simulink model "test_loopback_mux"  (Simulink 7.0)
settings: Solver=ode45  StartTime=0.0  StopTime=4000  RelTol=1e-3
libraries: xbsIndex_r4 x498, xps_library x21, xbsReplacements_r4 x18, casper_library x15
(part 2 of 3)

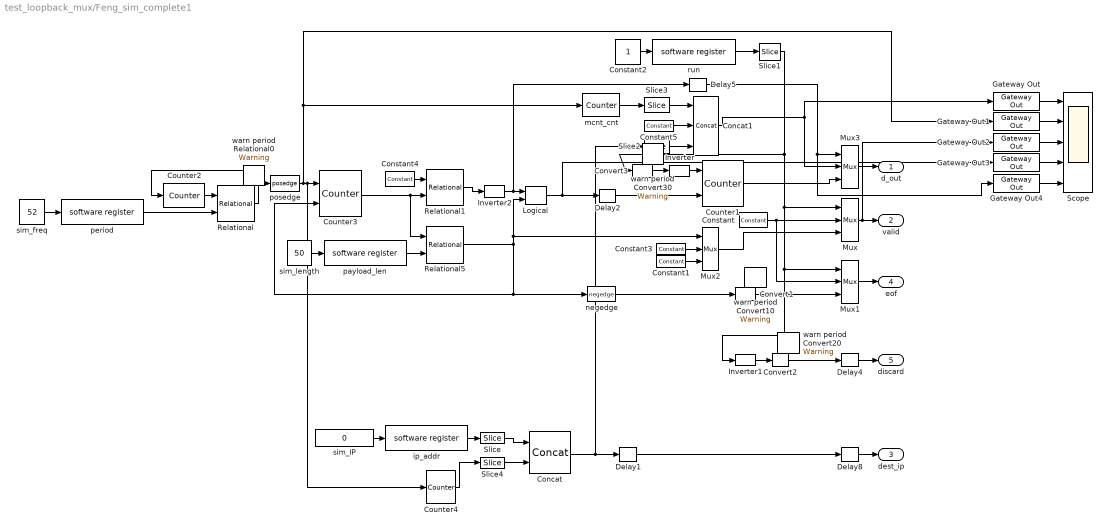
== system test_loopback_mux/Feng_sim_complete1 ==
  Concat : xbsIndex_r4/Concat  num_inputs=2  dbl_ovrd=off  block_type=concat
      settings: block_version=10.1.3
  Concat1 : xbsIndex_r4/Concat  num_inputs=3  dbl_ovrd=off  block_type=concat
      settings: block_version=10.1.3
  Constant : xbsIndex_r4/Constant  arith_type=Boolean  const=0  n_bits=1  bin_pt=0  explicit_period=on  period=1  equ=P=C  opselect=C  inp2=PCIN>>17  opr=+  inp1=P  carry=CIN  dbl_ovrd=off  block_type=constant
  Constant1 : xbsIndex_r4/Constant  arith_type=Boolean  const=1  n_bits=1  bin_pt=0  explicit_period=off  period=1  equ=P=C  opselect=C  inp2=PCIN>>17  opr=+  inp1=P  carry=CIN  dbl_ovrd=off  block_type=constant
  Constant2 : Constant  OutDataType=sfix(16)  OutScaling=2^0
  Constant3 : xbsIndex_r4/Constant  arith_type=Boolean  const=0  n_bits=1  bin_pt=0  explicit_period=off  period=1  equ=P=C  opselect=C  inp2=PCIN>>17  opr=+  inp1=P  carry=CIN  dbl_ovrd=off  block_type=constant
  Constant4 : xbsIndex_r4/Constant  arith_type=Unsigned  const=0  n_bits=32  bin_pt=0  explicit_period=on  period=1  equ=P=C  opselect=C  inp2=PCIN>>17  opr=+  inp1=P  carry=CIN  dbl_ovrd=off  block_type=constant
  Constant5 : xbsIndex_r4/Constant  arith_type=Unsigned  const=0  n_bits=16-2  bin_pt=0  explicit_period=on  period=1  equ=P=C  opselect=C  inp2=PCIN>>17  opr=+  inp1=P  carry=CIN  dbl_ovrd=off  block_type=constant
  Convert1 : xbsIndex_r4/Convert  arith_type=Boolean  n_bits=8  bin_pt=6  quantization=Truncate  overflow=Wrap  latency=0  dbl_ovrd=off  pipeline=off  block_type=convert
      settings: xl_area=[0, 0, 0, 0, 0, 0, 0]  block_version=10.1.3
  Convert2 : xbsIndex_r4/Convert  arith_type=Boolean  n_bits=8  bin_pt=6  quantization=Truncate  overflow=Wrap  latency=0  dbl_ovrd=off  pipeline=off  block_type=convert
      settings: xl_area=[0, 0, 0, 0, 0, 0, 0]  block_version=10.1.3
  Convert3 : xbsIndex_r4/Convert  arith_type=Boolean  n_bits=8  bin_pt=6  quantization=Truncate  overflow=Wrap  latency=0  dbl_ovrd=off  pipeline=off  block_type=convert
      settings: xl_area=[0, 0, 0, 0, 0, 0, 0]  block_version=10.1.3
  Counter1 : xbsIndex_r4/Counter  cnt_type=Free Running  cnt_to=Inf  operation=Up  start_count=0  cnt_by_val=1  arith_type=Unsigned  n_bits=64  bin_pt=0  load_pin=off  rst=on  en=on  explicit_period=off  period=1  dbl_ovrd=off  use_behavioral_HDL=off  use_rpm=off  implementation=Fabric  block_type=counter
      settings: xl_area=[0, 0, 0, 0, 0, 0, 0]
  Counter2 : xbsIndex_r4/Counter  cnt_type=Free Running  cnt_to=Inf  operation=Up  start_count=1  cnt_by_val=1  arith_type=Unsigned  n_bits=32  bin_pt=0  load_pin=off  rst=on  en=off  explicit_period=on  period=1  dbl_ovrd=off  use_behavioral_HDL=off  use_rpm=on  implementation=Fabric  block_type=counter
      settings: xl_area=[0, 0, 0, 0, 0, 0, 0]
  Counter3 : xbsIndex_r4/Counter  cnt_type=Free Running  cnt_to=1023  operation=Up  start_count=0  cnt_by_val=1  arith_type=Unsigned  n_bits=32  bin_pt=0  load_pin=off  rst=on  en=on  explicit_period=on  period=1  dbl_ovrd=off  use_behavioral_HDL=off  use_rpm=on  implementation=Fabric  block_type=counter
      settings: xl_area=[0, 0, 0, 0, 0, 0, 0]
  Counter4 : xbsIndex_r4/Counter  cnt_type=Free Running  cnt_to=1023  operation=Up  start_count=0  cnt_by_val=1  arith_type=Unsigned  n_bits=2  bin_pt=0  load_pin=off  rst=off  en=on  explicit_period=on  period=1  dbl_ovrd=off  use_behavioral_HDL=off  use_rpm=on  implementation=Fabric  block_type=counter
      settings: xl_area=[0, 0, 0, 0, 0, 0, 0]
  Delay{1..2,4..5,8} (5 alike) : xbsIndex_r4/Delay  en=off  latency=1  dbl_ovrd=off  reg_retiming=on  block_type=delay
      settings: xl_area=[0, 0, 0, 0, 0, 0, 0]
  Gateway Out{,1..4} (5 alike) : xbsIndex_r4/Gateway Out  hdl_port=on  timing_constraint=None  locs_specified=off  LOCs={}  block_type=gatewayout
      settings: infoedit="Gateway out block.  Converts Xilinx fixed point inputs into ouputs of type Simulink integer, double, or fixed point.<P><P>Hardware notes:  In hardware these blocks become top level output ports or are discarded, depending on how they are configured."  xl_area=[0, 0, 0, 0, 0, 0, 0]  block_version=10.1.3
  Inverter : xbsIndex_r4/Inverter  en=off  latency=0  dbl_ovrd=off  block_type=inv
      settings: xl_area=[0, 0, 0, 0, 0, 0, 0]
  Inverter1 : xbsIndex_r4/Inverter  en=off  latency=0  dbl_ovrd=off  block_type=inv
      settings: xl_area=[0, 0, 0, 0, 0, 0, 0]
  Inverter2 : xbsIndex_r4/Inverter  en=off  latency=0  dbl_ovrd=off  block_type=inv
      settings: xl_area=[0, 0, 0, 0, 0, 0, 0]
  Logical : xbsIndex_r4/Logical  logical_function=AND  inputs=2  en=off  latency=0  precision=Full  arith_type=Unsigned  n_bits=8  bin_pt=2  align_bp=on  dbl_ovrd=off  block_type=logical
      settings: xl_area=[0, 0, 0, 0, 0, 0, 0]
  Mux{,1..3} (4 alike) : xbsIndex_r4/Mux  inputs=2  en=off  latency=1  precision=Full  arith_type="Signed  (2's comp)"  n_bits=8  bin_pt=2  quantization=Truncate  overflow=Wrap  dbl_ovrd=off  block_type=mux
      settings: xl_area=[0, 0, 0, 0, 0, 0, 0]
  Relational : xbsIndex_r4/Relational  mode=a>=b  en=off  latency=0  dbl_ovrd=off  block_type=relational
      settings: xl_area=[0, 0, 0, 0, 0, 0, 0]  block_version=10.1.3
  Relational1 : xbsIndex_r4/Relational  mode=a=b  en=off  latency=0  dbl_ovrd=off  block_type=relational
      settings: xl_area=[0, 0, 0, 0, 0, 0, 0]  block_version=10.1.3
  Relational5 : xbsIndex_r4/Relational  mode=a<=b  en=off  latency=0  dbl_ovrd=off  block_type=relational
      settings: xl_area=[0, 0, 0, 0, 0, 0, 0]  block_version=10.1.3
  Scope : Scope  NumInputPorts=5
      settings: TimeRange=4000  YMin=130000~0~0~0~0  YMax=200000~1~1~1~1  SaveName=ScopeData11
  Slice : xbsIndex_r4/Slice  nbits=31  boolean_output=off  mode=Upper Bit Location + Width  bit1=0  base1=MSB of Input  bit0=0  base0=LSB of Input  dbl_ovrd=off  block_type=slice
      settings: infoedit="Extracts a given range of bits from each input sample and presents it at the output.  The output type is ordinarily unsigned with binary point at zero, but can be Boolean when the slice is one bit wide.<P><P>Hardware notes: In hardware this block costs nothing."  block_version=10.1.3
  Slice1 : xbsIndex_r4/Slice  nbits=1  boolean_output=off  mode=Lower Bit Location + Width  bit1=1  base1=MSB of Input  bit0=0  base0=LSB of Input  dbl_ovrd=off  block_type=slice
      settings: infoedit="Extracts a given range of bits from each input sample and presents it at the output.  The output type is ordinarily unsigned with binary point at zero, but can be Boolean when the slice is one bit wide.<P><P>Hardware notes: In hardware this block costs nothing."  block_version=10.1.3
  Slice2 : xbsIndex_r4/Slice  nbits=2  boolean_output=off  mode=Lower Bit Location + Width  bit1=1  base1=MSB of Input  bit0=0  base0=LSB of Input  dbl_ovrd=off  block_type=slice
      settings: infoedit="Extracts a given range of bits from each input sample and presents it at the output.  The output type is ordinarily unsigned with binary point at zero, but can be Boolean when the slice is one bit wide.<P><P>Hardware notes: In hardware this block costs nothing."  block_version=10.1.3
  Slice3 : xbsIndex_r4/Slice  nbits=48  boolean_output=off  mode=Lower Bit Location + Width  bit1=1  base1=MSB of Input  bit0=3  base0=LSB of Input  dbl_ovrd=off  block_type=slice
      settings: infoedit="Extracts a given range of bits from each input sample and presents it at the output.  The output type is ordinarily unsigned with binary point at zero, but can be Boolean when the slice is one bit wide.<P><P>Hardware notes: In hardware this block costs nothing."  block_version=10.1.3
  Slice4 : xbsIndex_r4/Slice  nbits=1  boolean_output=off  mode=Lower Bit Location + Width  bit1=1  base1=MSB of Input  bit0=1  base0=LSB of Input  dbl_ovrd=off  block_type=slice
      settings: infoedit="Extracts a given range of bits from each input sample and presents it at the output.  The output type is ordinarily unsigned with binary point at zero, but can be Boolean when the slice is one bit wide.<P><P>Hardware notes: In hardware this block costs nothing."  block_version=10.1.3
  ip_addr : xps_library/software register  Tag=xps:sw_reg  SystemSampleTime=-1  io_dir=From Processor  arith_type=Unsigned  bitwidth=32  bin_pt=0  sample_period=1  gw_name=test_loopback_mux_Feng_sim_complete1_ip_addr_user_data_out
      link override test_loopback_mux_Feng_sim_complete1_ip_addr_user_data_out: arith_type=Unsigned  n_bits=32  bin_pt=0  period=1
  mcnt_cnt : xbsIndex_r4/Counter  cnt_type=Free Running  cnt_to=Inf  operation=Up  start_count=0  cnt_by_val=1  arith_type=Unsigned  n_bits=64  bin_pt=0  load_pin=off  rst=off  en=on  explicit_period=off  period=1  dbl_ovrd=off  use_behavioral_HDL=off  use_rpm=off  implementation=Fabric  block_type=counter
      settings: xl_area=[0, 0, 0, 0, 0, 0, 0]
  negedge : casper_library/Misc/negedge  Tag=Rising Edge Detector  SystemSampleTime=-1
  payload_len : xps_library/software register  Tag=xps:sw_reg  SystemSampleTime=-1  io_dir=From Processor  arith_type=Unsigned  bitwidth=32  bin_pt=0  sample_period=1  gw_name=test_loopback_mux_Feng_sim_complete1_payload_len_user_data_out
      link override test_loopback_mux_Feng_sim_complete1_payload_len_user_data_out: arith_type=Unsigned  n_bits=32  bin_pt=0  period=1
  period : xps_library/software register  Tag=xps:sw_reg  SystemSampleTime=-1  io_dir=From Processor  arith_type=Unsigned  bitwidth=32  bin_pt=0  sample_period=1  gw_name=test_loopback_mux_Feng_sim_complete1_period_user_data_out
      link override test_loopback_mux_Feng_sim_complete1_period_user_data_out: arith_type=Unsigned  n_bits=32  bin_pt=0  period=1
  posedge : casper_library/Misc/pulse_ext/posedge  Tag=Rising Edge Detector  SystemSampleTime=-1
  run : xps_library/software register  Tag=xps:sw_reg  SystemSampleTime=-1  io_dir=From Processor  arith_type=Unsigned  bitwidth=32  bin_pt=0  sample_period=1  gw_name=test_loopback_mux_Feng_sim_complete1_run_user_data_out
      link override test_loopback_mux_Feng_sim_complete1_run_user_data_out: arith_type=Unsigned  n_bits=32  bin_pt=0  period=1
  sim_IP : Constant  Value=0  OutDataType=sfix(16)  OutScaling=2^0
  sim_freq : Constant  Value=52  OutDataType=sfix(16)  OutScaling=2^0
  sim_length : Constant  Value=50  OutDataType=sfix(16)  OutScaling=2^0
  warn period Convert10 : xbsReplacements_r4/Warning  SystemSampleTime=-1  period=1
  warn period Convert20 : xbsReplacements_r4/Warning  SystemSampleTime=-1  period=1
  warn period Convert30 : xbsReplacements_r4/Warning  SystemSampleTime=-1  period=1
  warn period Relational0 : xbsReplacements_r4/Warning  SystemSampleTime=-1  period=1
  d_out : Outport  OutDataType=sfix(16)  OutScaling=2^0
  valid : Outport  Port=2  OutDataType=sfix(16)  OutScaling=2^0
  dest_ip : Outport  Port=3  OutDataType=sfix(16)  OutScaling=2^0
  eof : Outport  Port=4  OutDataType=sfix(16)  OutScaling=2^0
  discard : Outport  Port=5  OutDataType=sfix(16)  OutScaling=2^0
  wires:
  Delay1/1 -> Delay8/1
  Slice2/1 -> Concat1/3
  Slice3/1 -> Concat1/1
  Logical/1 -> Gateway Out3/1, Delay2/1
  Gateway Out4/1 -> Scope/5
  Gateway Out3/1 -> Scope/4
  Gateway Out2/1 -> Scope/3
  Gateway Out1/1 -> Scope/2
  Gateway Out/1 -> Scope/1
  Delay5/1 -> Gateway Out4/1, Mux3/1
  Concat1/1 -> Gateway Out/1, Mux3/2
  Constant5/1 -> Concat1/2
  mcnt_cnt/1 -> Slice3/1
  Inverter2/1 -> Logical/1, Delay5/1
  Relational1/1 -> Inverter2/1
  Constant4/1 -> Relational1/1
  Concat/1 -> Slice2/1, Delay1/1
  Slice/1 -> Concat/1
  Counter4/1 -> Slice4/1
  ip_addr/1 -> Slice/1
  Convert2/1 -> Delay4/1
  Inverter1/1 -> Convert2/1
  Constant1/1 -> Mux2/3
  Constant3/1 -> Mux2/2
  Convert3/1 -> Inverter/1
  Delay2/1 -> Counter1/2
  Inverter/1 -> Counter1/1
  Mux2/1 -> Mux/3
  Delay4/1 -> discard/1
  Slice1/1 -> Convert3/1, Inverter1/1, Mux1/1, Mux/1
  Constant2/1 -> run/1
  run/1 -> Slice1/1
  Delay8/1 -> dest_ip/1
  Mux3/1 -> d_out/1
  Convert1/1 -> Mux1/3
  Mux1/1 -> eof/1
  Constant/1 -> Mux1/2, Mux/2
  Mux/1 -> Gateway Out2/1, valid/1
  payload_len/1 -> Relational5/2
  sim_length/1 -> payload_len/1
  posedge/1 -> Gateway Out1/1, mcnt_cnt/1, Counter4/1, Counter3/1
  Counter3/1 -> Relational1/2, Relational5/1
  Relational5/1 -> Counter3/2, negedge/1, Mux2/1, Logical/2
  sim_IP/1 -> ip_addr/1
  sim_freq/1 -> period/1
  period/1 -> Relational/2
  negedge/1 -> Convert1/1
  Counter1/1 -> Mux3/3
  Relational/1 -> Counter2/1, posedge/1
  Counter2/1 -> Relational/1
  Slice4/1 -> Concat/2

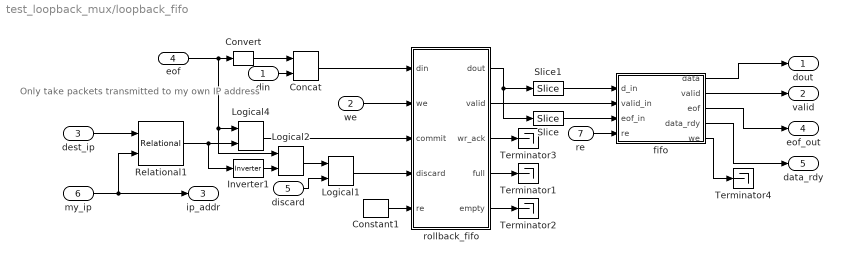
== system test_loopback_mux/loopback_fifo ==
  note: Only take packets transmitted
      | to my own IP address
  din : Inport  OutDataType=sfix(16)  OutScaling=2^0
  we : Inport  Port=2  OutDataType=sfix(16)  OutScaling=2^0
  dest_ip : Inport  Port=3  OutDataType=sfix(16)  OutScaling=2^0
  eof : Inport  Port=4  OutDataType=sfix(16)  OutScaling=2^0
  discard : Inport  Port=5  OutDataType=sfix(16)  OutScaling=2^0
  my_ip : Inport  Port=6  OutDataType=sfix(16)  OutScaling=2^0
  re : Inport  Port=7  OutDataType=sfix(16)  OutScaling=2^0
  Concat : xbsIndex_r4/Concat  num_inputs=2  dbl_ovrd=off  block_type=concat
      settings: block_version=10.1.3
  Constant1 : xbsIndex_r4/Constant  arith_type=Boolean  const=1  n_bits=2  bin_pt=0  explicit_period=on  period=1  equ=P=C  opselect=C  inp2=PCIN>>17  opr=+  inp1=P  carry=CIN  dbl_ovrd=off  block_type=constant
  Convert : xbsIndex_r4/Convert  arith_type=Unsigned  n_bits=1  bin_pt=0  quantization=Truncate  overflow=Wrap  latency=0  dbl_ovrd=off  pipeline=off  block_type=convert
      settings: xl_area=[0, 0, 0, 0, 0, 0, 0]  block_version=10.1.3
  Inverter1 : xbsIndex_r4/Inverter  en=off  latency=0  dbl_ovrd=off  block_type=inv
      settings: xl_area=[0, 0, 0, 0, 0, 0, 0]
  Logical1 : xbsIndex_r4/Logical  logical_function=OR  inputs=2  en=off  latency=0  precision=Full  arith_type=Unsigned  n_bits=8  bin_pt=2  align_bp=on  dbl_ovrd=off  block_type=logical
      settings: xl_area=[0, 0, 0, 0, 0, 0, 0]
  Logical2 : xbsIndex_r4/Logical  logical_function=AND  inputs=2  en=off  latency=0  precision=Full  arith_type=Unsigned  n_bits=8  bin_pt=2  align_bp=on  dbl_ovrd=off  block_type=logical
      settings: xl_area=[0, 0, 0, 0, 0, 0, 0]
  Logical4 : xbsIndex_r4/Logical  logical_function=AND  inputs=2  en=off  latency=0  precision=Full  arith_type=Unsigned  n_bits=8  bin_pt=2  align_bp=on  dbl_ovrd=off  block_type=logical
      settings: xl_area=[0, 0, 0, 0, 0, 0, 0]
  Relational1 : xbsIndex_r4/Relational  mode=a=b  en=off  latency=1  dbl_ovrd=off  block_type=relational
      settings: xl_area=[0, 0, 0, 0, 0, 0, 0]  block_version=10.1.3
  Slice : xbsIndex_r4/Slice  nbits=1  boolean_output=on  mode=Upper Bit Location + Width  bit1=0  base1=MSB of Input  bit0=0  base0=LSB of Input  dbl_ovrd=off  block_type=slice
      settings: infoedit="Extracts a given range of bits from each input sample and presents it at the output.  The output type is ordinarily unsigned with binary point at zero, but can be Boolean when the slice is one bit wide.<P><P>Hardware notes: In hardware this block costs nothing."  block_version=10.1.3
  Slice1 : xbsIndex_r4/Slice  nbits=64  boolean_output=off  mode=Lower Bit Location + Width  bit1=-1  base1=MSB of Input  bit0=0  base0=LSB of Input  dbl_ovrd=off  block_type=slice
      settings: infoedit="Extracts a given range of bits from each input sample and presents it at the output.  The output type is ordinarily unsigned with binary point at zero, but can be Boolean when the slice is one bit wide.<P><P>Hardware notes: In hardware this block costs nothing."  block_version=10.1.3
  Terminator{1..4} (4 alike) : Terminator
  fifo : Subsystem
  rollback_fifo : Subsystem  mask{depth_bits=7}
      mask prompts: depth_bits "Fifo Depth (2^?):"
      mask help: A rollback fifo behaves as a normal fifo, except that data which are written in have to be "committed" before they become available for readout. Moreover, any data which are written in and have not been committed can be "discarded", and will never be made available for readout.
  dout : Outport  OutDataType=sfix(16)  OutScaling=2^0
  valid : Outport  Port=2  OutDataType=sfix(16)  OutScaling=2^0
  ip_addr : Outport  Port=3  OutDataType=sfix(16)  OutScaling=2^0
  eof_out : Outport  Port=4  OutDataType=sfix(16)  OutScaling=2^0
  data_rdy : Outport  Port=5  OutDataType=sfix(16)  OutScaling=2^0
  wires:
  Logical2/1 -> Logical1/1
  Inverter1/1 -> Logical2/2
  discard/1 -> Logical1/2
  Logical1/1 -> rollback_fifo/4(discard)
  Convert/1 -> Concat/1
  din/1 -> Concat/2
  Concat/1 -> rollback_fifo/1(din)
  Logical4/1 -> rollback_fifo/3(commit)
  we/1 -> rollback_fifo/2(we)
  eof/1 -> Logical2/1, Logical4/1, Convert/1
  Relational1/1 -> Inverter1/1, Logical4/2
  dest_ip/1 -> Relational1/1
  Constant1/1 -> rollback_fifo/5(re)
  rollback_fifo/2(valid) -> fifo/2(valid_in)
  re/1 -> fifo/4(re)
  fifo/2(valid) -> valid/1
  fifo/3(eof) -> eof_out/1
  fifo/1(data) -> dout/1
  fifo/4(data_rdy) -> data_rdy/1
  my_ip/1 -> Relational1/2, ip_addr/1
  Slice1/1 -> fifo/1(d_in)
  rollback_fifo/1(dout) -> Slice1/1, Slice/1
  Slice/1 -> fifo/3(eof_in)
  rollback_fifo/5(empty) -> Terminator2/1
  rollback_fifo/4(full) -> Terminator1/1
  rollback_fifo/3(wr_ack) -> Terminator3/1
  fifo/5(we) -> Terminator4/1

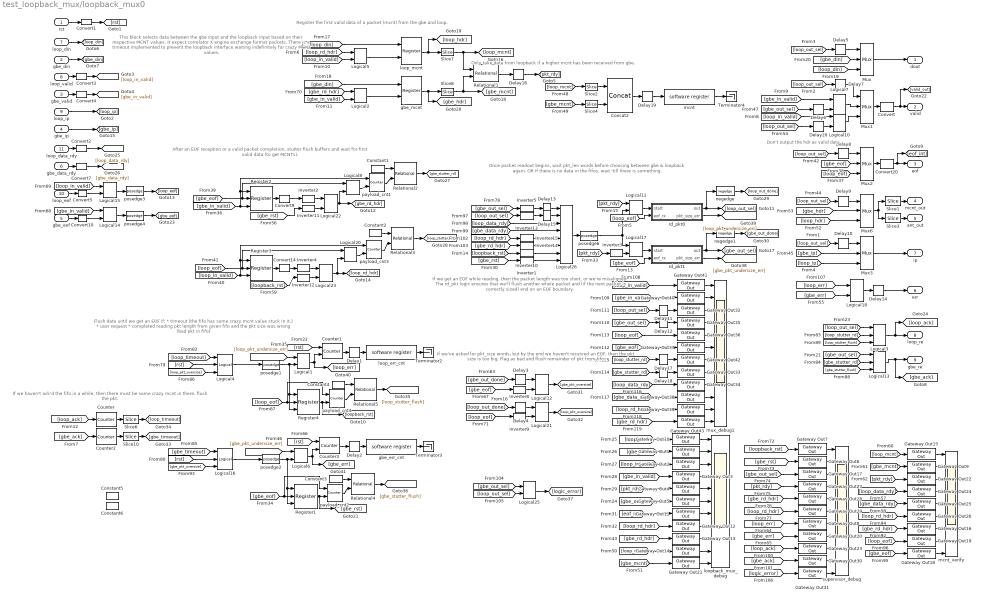
== system test_loopback_mux/loopback_mux0 ==
  note: Once packet readout begins, wait pkt_len words
      | before choosing between gbe & loopback again.
      | OR
      | If there is no data in the fifos, wait 'till there is something.
  note: Only take data from loopback
      | if a higher mcnt has been
      | received from gbe.
  note: This block selects data between the gbe input
      | and the loopback input based on their respective MCNT values.
      | It expect correlator X engine exchange format packets.
      |
      | There is a timeout implemented to prevent the loopback interface
      | waiting indefinitely for crazy MCNT values.
  note: Don't output the hdr as valid data
  note: Register the first valid
      | data of a packet (mcnt)
      | from the gbe and loop.
  note: After an EOF reception or a valid packet completion,
      |  stutter flush buffers and wait for first valid data (to get MCNTs).
  note: Flush data until we get an EOF if:
      |  * timeout (the fifo has some crazy mcnt value stuck in it.)
      |  * user request
      |  * completed reading pkt length from given fifo and the pkt size was wrong (bad pkt in fifo)
  note: If we've asked for pkt_size words,
      | but by the end we haven't received an EOF,
      | then the pkt size is too big.
      | Flag as bad and flush remainder of pkt from fifo.
  note: If we haven't ack'd the fifo in a while,
      | then there must be some crazy mcnt in there.
      | flush the pkt.
  note: If we get an EOF while reading,
      | then the packet length was too short, or we're misaligned.
      | The rd_pkt logic ensures that we'll flush another whole packet and
      | (if the next packet is correctly sized) end on an EOF boundary.
  rst : Inport  OutDataType=sfix(16)  OutScaling=2^0
  gbe_din : Inport  Port=2  OutDataType=sfix(16)  OutScaling=2^0
  gbe_valid : Inport  Port=3  OutDataType=sfix(16)  OutScaling=2^0
  gbe_ip : Inport  Port=4  OutDataType=sfix(16)  OutScaling=2^0
  gbe_eof : Inport  Port=5  OutDataType=sfix(16)  OutScaling=2^0
  gbe_data_rdy : Inport  Port=6  OutDataType=sfix(16)  OutScaling=2^0
  loop_din : Inport  Port=7  OutDataType=sfix(16)  OutScaling=2^0
  loop_valid : Inport  Port=8  OutDataType=sfix(16)  OutScaling=2^0
  loop_ip : Inport  Port=9  OutDataType=sfix(16)  OutScaling=2^0
  loop_eof : Inport  Port=10  OutDataType=sfix(16)  OutScaling=2^0
  loop_data_rdy : Inport  Port=11  OutDataType=sfix(16)  OutScaling=2^0
  Concat2 : xbsIndex_r4/Concat  num_inputs=2  dbl_ovrd=off  block_type=concat
      settings: block_version=10.1.3
  Constant{1..4} (4 alike) : xbsIndex_r4/Constant  arith_type=Unsigned  const=1  n_bits=ceil(log2(fifo_latency))  bin_pt=0  explicit_period=on  period=1  equ=P=C  opselect=C  inp2=PCIN>>17  opr=+  inp1=P  carry=CIN  dbl_ovrd=off  block_type=constant
  Constant5 : xbsIndex_r4/Constant  arith_type=Boolean  const=0  n_bits=ceil(log2(fifo_latency))  bin_pt=0  explicit_period=on  period=1  equ=P=C  opselect=C  inp2=PCIN>>17  opr=+  inp1=P  carry=CIN  dbl_ovrd=off  block_type=constant
  Constant6 : xbsIndex_r4/Constant  arith_type=Boolean  const=0  n_bits=ceil(log2(fifo_latency))  bin_pt=0  explicit_period=on  period=1  equ=P=C  opselect=C  inp2=PCIN>>17  opr=+  inp1=P  carry=CIN  dbl_ovrd=off  block_type=constant
  Convert{,1,9,14,20} (5 alike) : xbsIndex_r4/Convert  arith_type=Boolean  n_bits=8  bin_pt=6  quantization=Truncate  overflow=Wrap  latency=0  dbl_ovrd=off  pipeline=off  block_type=convert
      settings: xl_area=[0, 0, 0, 0, 0, 0, 0]  block_version=10.1.3
  Convert{2..5,7,10} (6 alike) : xbsIndex_r4/Convert  arith_type=Boolean  n_bits=1  bin_pt=0  quantization=Truncate  overflow=Wrap  latency=0  dbl_ovrd=off  pipeline=off  block_type=convert
      settings: xl_area=[0, 0, 0, 0, 0, 0, 0]  block_version=10.1.3
  Counter : xbsIndex_r4/Counter  cnt_type=Free Running  cnt_to=Inf  operation=Up  start_count=0  cnt_by_val=1  arith_type=Unsigned  n_bits=timeout_bits+1  bin_pt=0  load_pin=off  rst=on  en=off  explicit_period=off  period=1  dbl_ovrd=off  use_behavioral_HDL=off  use_rpm=on  implementation=Fabric  block_type=counter
      settings: xl_area=[0, 0, 0, 0, 0, 0, 0]
  Counter1 : xbsIndex_r4/Counter  cnt_type=Free Running  cnt_to=Inf  operation=Up  start_count=0  cnt_by_val=1  arith_type=Unsigned  n_bits=27  bin_pt=0  load_pin=off  rst=on  en=on  explicit_period=off  period=1  dbl_ovrd=off  use_behavioral_HDL=off  use_rpm=on  implementation=Fabric  block_type=counter
      settings: xl_area=[0, 0, 0, 0, 0, 0, 0]
  Counter2 : xbsIndex_r4/Counter  cnt_type=Free Running  cnt_to=Inf  operation=Up  start_count=0  cnt_by_val=1  arith_type=Unsigned  n_bits=timeout_bits+1  bin_pt=0  load_pin=off  rst=on  en=off  explicit_period=off  period=1  dbl_ovrd=off  use_behavioral_HDL=off  use_rpm=on  implementation=Fabric  block_type=counter
      settings: xl_area=[0, 0, 0, 0, 0, 0, 0]
  Counter3 : xbsIndex_r4/Counter  cnt_type=Free Running  cnt_to=Inf  operation=Up  start_count=0  cnt_by_val=1  arith_type=Unsigned  n_bits=27  bin_pt=0  load_pin=off  rst=on  en=on  explicit_period=off  period=1  dbl_ovrd=off  use_behavioral_HDL=off  use_rpm=on  implementation=Fabric  block_type=counter
      settings: xl_area=[0, 0, 0, 0, 0, 0, 0]
  Delay{1..2,14,19} (4 alike) : xbsIndex_r4/Delay  en=off  latency=2  dbl_ovrd=off  reg_retiming=on  block_type=delay
      settings: xl_area=[0, 0, 0, 0, 0, 0, 0]
  Delay{5..13,15,17..18,20} (13 alike) : xbsIndex_r4/Delay  en=off  latency=fifo_latency  dbl_ovrd=off  reg_retiming=on  block_type=delay
      settings: xl_area=[0, 0, 0, 0, 0, 0, 0]
  Delay16 : xbsIndex_r4/Delay  en=off  latency=1  dbl_ovrd=off  reg_retiming=on  block_type=delay
      settings: xl_area=[0, 0, 0, 0, 0, 0, 0]
  Delay3 : xbsIndex_r4/Delay  en=off  latency=fifo_latency-1  dbl_ovrd=off  reg_retiming=on  block_type=delay
      settings: xl_area=[0, 0, 0, 0, 0, 0, 0]
  Delay4 : xbsIndex_r4/Delay  en=off  latency=fifo_latency-1  dbl_ovrd=off  reg_retiming=on  block_type=delay
      settings: xl_area=[0, 0, 0, 0, 0, 0, 0]
  Gateway Out{1..43} (43 alike) : xbsIndex_r4/Gateway Out  hdl_port=off  timing_constraint=None  locs_specified=off  LOCs={}  block_type=gatewayout
      settings: infoedit="Gateway out block.  Converts Xilinx fixed point inputs into ouputs of type Simulink integer, double, or fixed point.<P><P>Hardware notes:  In hardware these blocks become top level output ports or are discarded, depending on how they are configured."  xl_area=[0, 0, 0, 0, 0, 0, 0]  block_version=10.1.3
  Inverter{1..5,8..15} (13 alike) : xbsIndex_r4/Inverter  en=off  latency=0  dbl_ovrd=off  block_type=inv
      settings: xl_area=[0, 0, 0, 0, 0, 0, 0]
  Logical{1,6,8,18,20} (5 alike) : xbsIndex_r4/Logical  logical_function=OR  inputs=2  en=off  latency=0  precision=Full  arith_type=Unsigned  n_bits=8  bin_pt=2  align_bp=on  dbl_ovrd=off  block_type=logical
      settings: xl_area=[0, 0, 0, 0, 0, 0, 0]
  Logical{2,5,7,10..12,14..15,17,21..23,25} (13 alike) : xbsIndex_r4/Logical  logical_function=AND  inputs=2  en=off  latency=0  precision=Full  arith_type=Unsigned  n_bits=8  bin_pt=2  align_bp=on  dbl_ovrd=off  block_type=logical
      settings: xl_area=[0, 0, 0, 0, 0, 0, 0]
  Logical{3..4,13,16} (4 alike) : xbsIndex_r4/Logical  logical_function=OR  inputs=3  en=off  latency=0  precision=Full  arith_type=Unsigned  n_bits=8  bin_pt=2  align_bp=on  dbl_ovrd=off  block_type=logical
      settings: xl_area=[0, 0, 0, 0, 0, 0, 0]
  Logical26 : xbsIndex_r4/Logical  logical_function=AND  inputs=8  en=off  latency=0  precision=Full  arith_type=Unsigned  n_bits=8  bin_pt=2  align_bp=on  dbl_ovrd=off  block_type=logical
      settings: xl_area=[0, 0, 0, 0, 0, 0, 0]
  Mux{,1..3,6} (5 alike) : xbsIndex_r4/Mux  inputs=2  en=off  latency=0  precision=Full  arith_type="Signed  (2's comp)"  n_bits=8  bin_pt=2  quantization=Truncate  overflow=Wrap  dbl_ovrd=off  block_type=mux
      settings: xl_area=[0, 0, 0, 0, 0, 0, 0]
  Register{1..4} (4 alike) : xbsIndex_r4/Register  init=0  rst=on  en=on  dbl_ovrd=off  block_type=register
      settings: xl_area=[0, 0, 0, 0, 0, 0, 0]
  Relational1 : xbsIndex_r4/Relational  mode=a<b  en=off  latency=1  dbl_ovrd=off  block_type=relational
      settings: xl_area=[0, 0, 0, 0, 0, 0, 0]  block_version=10.1.3
  Relational{2..5} (4 alike) : xbsIndex_r4/Relational  mode=a=b  en=off  latency=0  dbl_ovrd=off  block_type=relational
      settings: xl_area=[0, 0, 0, 0, 0, 0, 0]  block_version=10.1.3
  Slice1 : xbsIndex_r4/Slice  nbits=48  boolean_output=off  mode=Lower Bit Location + Width  bit1=0  base1=MSB of Input  bit0=16  base0=LSB of Input  dbl_ovrd=off  block_type=slice
      settings: infoedit="Extracts a given range of bits from each input sample and presents it at the output.  The output type is ordinarily unsigned with binary point at zero, but can be Boolean when the slice is one bit wide.<P><P>Hardware notes: In hardware this block costs nothing."  block_version=10.1.3
  Slice10 : xbsIndex_r4/Slice  nbits=1  boolean_output=on  mode=Upper Bit Location + Width  bit1=0  base1=MSB of Input  bit0=1  base0=LSB of Input  dbl_ovrd=off  block_type=slice
      settings: infoedit="Extracts a given range of bits from each input sample and presents it at the output.  The output type is ordinarily unsigned with binary point at zero, but can be Boolean when the slice is one bit wide.<P><P>Hardware notes: In hardware this block costs nothing."  block_version=10.1.3
  Slice2 : xbsIndex_r4/Slice  nbits=16  boolean_output=off  mode=Lower Bit Location + Width  bit1=0  base1=MSB of Input  bit0=0  base0=LSB of Input  dbl_ovrd=off  block_type=slice
      settings: infoedit="Extracts a given range of bits from each input sample and presents it at the output.  The output type is ordinarily unsigned with binary point at zero, but can be Boolean when the slice is one bit wide.<P><P>Hardware notes: In hardware this block costs nothing."  block_version=10.1.3
  Slice3 : xbsIndex_r4/Slice  nbits=16  boolean_output=off  mode=Lower Bit Location + Width  bit1=0  base1=MSB of Input  bit0=0  base0=LSB of Input  dbl_ovrd=off  block_type=slice
      settings: infoedit="Extracts a given range of bits from each input sample and presents it at the output.  The output type is ordinarily unsigned with binary point at zero, but can be Boolean when the slice is one bit wide.<P><P>Hardware notes: In hardware this block costs nothing."  block_version=10.1.3
  Slice4 : xbsIndex_r4/Slice  nbits=16  boolean_output=off  mode=Lower Bit Location + Width  bit1=0  base1=MSB of Input  bit0=0  base0=LSB of Input  dbl_ovrd=off  block_type=slice
      settings: infoedit="Extracts a given range of bits from each input sample and presents it at the output.  The output type is ordinarily unsigned with binary point at zero, but can be Boolean when the slice is one bit wide.<P><P>Hardware notes: In hardware this block costs nothing."  block_version=10.1.3
  Slice6 : xbsIndex_r4/Slice  nbits=1  boolean_output=on  mode=Upper Bit Location + Width  bit1=0  base1=MSB of Input  bit0=1  base0=LSB of Input  dbl_ovrd=off  block_type=slice
      settings: infoedit="Extracts a given range of bits from each input sample and presents it at the output.  The output type is ordinarily unsigned with binary point at zero, but can be Boolean when the slice is one bit wide.<P><P>Hardware notes: In hardware this block costs nothing."  block_version=10.1.3
  Slice7 : xbsIndex_r4/Slice  nbits=48  boolean_output=off  mode=Upper Bit Location + Width  bit1=0  base1=MSB of Input  bit0=0  base0=LSB of Input  dbl_ovrd=off  block_type=slice
      settings: infoedit="Extracts a given range of bits from each input sample and presents it at the output.  The output type is ordinarily unsigned with binary point at zero, but can be Boolean when the slice is one bit wide.<P><P>Hardware notes: In hardware this block costs nothing."  block_version=10.1.3
  Slice8 : xbsIndex_r4/Slice  nbits=48  boolean_output=off  mode=Upper Bit Location + Width  bit1=0  base1=MSB of Input  bit0=0  base0=LSB of Input  dbl_ovrd=off  block_type=slice
      settings: infoedit="Extracts a given range of bits from each input sample and presents it at the output.  The output type is ordinarily unsigned with binary point at zero, but can be Boolean when the slice is one bit wide.<P><P>Hardware notes: In hardware this block costs nothing."  block_version=10.1.3
  Terminator2 : Terminator
  Terminator3 : Terminator
  Terminator4 : Terminator
  gbe_err_cnt : xps_library/software register  Tag=xps:sw_reg  SystemSampleTime=-1  io_dir=To Processor  arith_type=Unsigned  bitwidth=32  bin_pt=0  sample_period=1  gw_name=test_loopback_mux_loopback_mux0_gbe_err_cnt_user_data_in
      link override convert: arith_type=Unsigned  n_bits=32  bin_pt=0
  gbe_mcnt : xbsIndex_r4/Register  init=0  rst=off  en=on  dbl_ovrd=off  block_type=register
      settings: xl_area=[0, 0, 0, 0, 0, 0, 0]
  loop_err_cnt : xps_library/software register  Tag=xps:sw_reg  SystemSampleTime=-1  io_dir=To Processor  arith_type=Unsigned  bitwidth=32  bin_pt=0  sample_period=1  gw_name=test_loopback_mux_loopback_mux0_loop_err_cnt_user_data_in
      link override convert: arith_type=Unsigned  n_bits=32  bin_pt=0
  loop_mcnt : xbsIndex_r4/Register  init=0  rst=off  en=on  dbl_ovrd=off  block_type=register
      settings: xl_area=[0, 0, 0, 0, 0, 0, 0]
  loopback_mux_debug : Scope  NumInputPorts=11
      settings: YMin=300~190.95~0~0.95~0.95~-1~-1~-1~-5~-5~-5  YMax=525~211.05~1~1.05~1.05~1~1~1~5~5~5  SaveName=ScopeData7
  mcnt : xps_library/software register  Tag=xps:sw_reg  SystemSampleTime=-1  io_dir=To Processor  arith_type=Unsigned  bitwidth=32  bin_pt=0  sample_period=1  gw_name=test_loopback_mux_loopback_mux0_mcnt_user_data_in
      link override convert: arith_type=Unsigned  n_bits=32  bin_pt=0
  mcnt_verify : Scope  NumInputPorts=9
      settings: YMin=300~190.95~0~-5~-5~-5~-5~-5~-5  YMax=525~211.05~1~5~5~5~5~5~5  SaveName=ScopeData2
  mux_debug1 : Scope  NumInputPorts=12
      settings: YMin=300~190.95~0~-5~-5~-5~-5~-5~-5~-5~-5~-5  YMax=525~211.05~1~5~5~5~5~5~5~5~5~5  SaveName=ScopeData3
  negedge : casper_library/Misc/negedge  Tag=Rising Edge Detector  SystemSampleTime=-1
  negedge1 : casper_library/Misc/negedge  Tag=Rising Edge Detector  SystemSampleTime=-1
  payload_cnt{1..4} (4 alike) : xbsIndex_r4/Counter  cnt_type=Count Limited  cnt_to=max((fifo_latency + 1),2)  operation=Up  start_count=0  cnt_by_val=1  arith_type=Unsigned  n_bits=ceil(log2(fifo_latency))+1  bin_pt=0  load_pin=off  rst=on  en=on  explicit_period=on  period=1  dbl_ovrd=off  use_behavioral_HDL=off  use_rpm=on  implementation=Fabric  block_type=counter
      settings: xl_area=[0, 0, 0, 0, 0, 0, 0]
  posedge{1..4,6} (5 alike) : casper_library/Misc/posedge  Tag=Rising Edge Detector  SystemSampleTime=-1
  rd_pkt0 : Subsystem
  rd_pkt1 : Subsystem
  supervisor_debug : Scope  NumInputPorts=11
      settings: YMin=300~190.95~0~-5~-5~-5~-5~-5~-5~-5~-5  YMax=525~211.05~1~5~5~5~5~5~5~5~5  SaveName=ScopeData18
  dout : Outport  OutDataType=sfix(16)  OutScaling=2^0
  valid : Outport  Port=2  OutDataType=sfix(16)  OutScaling=2^0
  eof : Outport  Port=3  OutDataType=sfix(16)  OutScaling=2^0
  mcnt_out : Outport  Port=4  OutDataType=sfix(16)  OutScaling=2^0
  ant_out : Outport  Port=5  OutDataType=sfix(16)  OutScaling=2^0
  err : Outport  Port=6  OutDataType=sfix(16)  OutScaling=2^0
  ip : Outport  Port=7  OutDataType=sfix(16)  OutScaling=2^0
  loop_re : Outport  Port=8  OutDataType=sfix(16)  OutScaling=2^0
  gbe_re : Outport  Port=9  OutDataType=sfix(16)  OutScaling=2^0
  wires:
  Mux/1 -> dout/1
  Mux1/1 -> Convert/1
  Mux2/1 -> Convert20/1
  gbe_valid/1 -> Convert4/1
  loop_valid/1 -> Convert3/1
  Convert/1 -> valid/1, [valid_out]
  Slice2/1 -> Concat2/1
  Slice4/1 -> Concat2/2
  Concat2/1 -> Delay19/1
  Delay5/1 -> Mux/1
  [loop_out_sel] -> Delay5/1
  [loop_out_sel] -> Delay8/1
  Gateway Out2/1 -> loopback_mux_debug/3
  Gateway Out3/1 -> loopback_mux_debug/4
  Gateway Out4/1 -> loopback_mux_debug/5
  Gateway Out5/1 -> loopback_mux_debug/6
  Convert3/1 -> [loop_in_valid]
  Convert4/1 -> [gbe_in_valid]
  Relational1/1 -> Delay16/1
  loop_din/1 -> [loop_din]
  gbe_din/1 -> [gbe_din]
  [gbe_din] -> Gateway Out1/1
  [loop_din] -> Gateway Out10/1
  [loop_in_valid] -> Gateway Out2/1
  [gbe_in_valid] -> Gateway Out3/1
  [gbe_out_sel] -> Gateway Out5/1
  [pkt_rdy] -> Gateway Out4/1
  Gateway Out11/1 -> loopback_mux_debug/7
  [eof_int] -> Gateway Out11/1
  [loop_rd_hdr] -> Gateway Out12/1
  Gateway Out12/1 -> loopback_mux_debug/8
  loop_eof/1 -> Convert5/1
  gbe_eof/1 -> Convert10/1
  Gateway Out13/1 -> loopback_mux_debug/9
  [gbe_rd_hdr] -> Gateway Out13/1
  [loop_out_sel] -> Delay7/1
  loop_ip/1 -> [loop_ip]
  gbe_ip/1 -> [gbe_ip]
  Mux3/1 -> ip/1
  [loop_out_sel] -> Delay10/1
  [loop_mcnt] -> Slice2/1
  [gbe_mcnt] -> Slice4/1
  Gateway Out10/1 -> loopback_mux_debug/1
  Gateway Out1/1 -> loopback_mux_debug/2
  Gateway Out14/1 -> loopback_mux_debug/10
  Gateway Out21/1 -> loopback_mux_debug/11
  [loop_mcnt] -> Gateway Out14/1
  [gbe_mcnt] -> Gateway Out21/1
  Gateway Out22/1 -> mcnt_verify/3
  Gateway Out15/1 -> mcnt_verify/1
  Gateway Out9/1 -> mcnt_verify/2
  Gateway Out24/1 -> mcnt_verify/4
  Gateway Out25/1 -> mcnt_verify/5
  Gateway Out26/1 -> mcnt_verify/6
  Gateway Out16/1 -> mcnt_verify/7
  [loop_mcnt] -> Gateway Out15/1
  [gbe_mcnt] -> Gateway Out9/1
  [pkt_rdy] -> Gateway Out22/1
  Slice7/1 -> Relational1/1, [loop_mcnt]
  Slice8/1 -> Relational1/2, [gbe_mcnt]
  Slice1/1 -> mcnt_out/1
  Slice3/1 -> ant_out/1
  Mux6/1 -> Slice1/1, Slice3/1
  Counter2/1 -> Slice10/1
  [gbe_ack] -> Counter2/1
  [rst] -> Counter3/1
  Counter3/1 -> Delay2/1
  Logical16/1 -> posedge2/1
  Logical14/1 -> posedge4/1
  Logical15/1 -> posedge3/1
  Convert5/1 -> Logical15/2
  Convert10/1 -> Logical14/2
  [gbe_in_valid] -> Logical14/1
  [loop_in_valid] -> Logical15/1
  Gateway Out17/1 -> supervisor_debug/3
  Gateway Out7/1 -> supervisor_debug/1
  Gateway Out6/1 -> supervisor_debug/2
  Gateway Out27/1 -> supervisor_debug/4
  Gateway Out28/1 -> supervisor_debug/5
  Gateway Out29/1 -> supervisor_debug/6
  Gateway Out8/1 -> supervisor_debug/7
  [loopback_rst] -> Gateway Out7/1
  [gbe_rst] -> Gateway Out6/1
  [gbe_out_sel] -> Gateway Out17/1
  [pkt_rdy] -> Gateway Out27/1
  [gbe_rd_hdr] -> Gateway Out28/1
  [loop_rd_hdr] -> Gateway Out29/1
  Logical3/1 -> loop_re/1, [loop_ack]
  Logical13/1 -> gbe_re/1, [gbe_ack]
  rst/1 -> Convert1/1
  Delay14/1 -> err/1
  Logical18/1 -> Delay14/1
  Counter/1 -> Slice6/1
  [loop_ack] -> Counter/1
  [rst] -> Counter1/1
  Counter1/1 -> Delay1/1
  Logical4/1 -> posedge1/1
  [pkt_rdy] -> Logical11/1
  Register2/1 -> Convert9/1
  Logical22/1 -> [gbe_rd_hdr], Logical8/2
  Register3/1 -> Convert14/1
  Convert14/1 -> Inverter4/1
  gbe_mcnt/1 -> Slice8/1, [gbe_hdr]
  loop_mcnt/1 -> Slice7/1, [loop_hdr]
  Logical5/1 -> loop_mcnt/2
  [loop_rd_hdr] -> Logical5/1
  [gbe_rd_hdr] -> Logical2/1
  [loop_in_valid] -> Logical5/2
  [gbe_in_valid] -> Logical2/2
  [loop_din] -> loop_mcnt/1
  [gbe_din] -> gbe_mcnt/1
  Convert1/1 -> [rst]
  Convert20/1 -> [eof_int], eof/1
  posedge1/1 -> Register4/3, Register4/1, Logical1/2
  posedge2/1 -> Register1/1, Register1/3, Logical6/2
  posedge3/1 -> [loop_eof]
  posedge4/1 -> [gbe_eof]
  Delay1/1 -> loop_err_cnt/1
  Delay2/1 -> gbe_err_cnt/1
  Logical2/1 -> gbe_mcnt/2
  Delay16/1 -> [pkt_rdy]
  [loop_out_sel] -> Delay20/1
  Delay19/1 -> mcnt/1
  loop_err_cnt/1 -> Terminator2/1
  gbe_err_cnt/1 -> Terminator3/1
  mcnt/1 -> Terminator4/1
  gbe_data_rdy/1 -> Convert7/1
  loop_data_rdy/1 -> Convert2/1
  Convert2/1 -> [loop_data_rdy]
  Convert7/1 -> [gbe_data_rdy]
  payload_cnt1/1 -> Relational2/2
  Constant1/1 -> Relational2/1
  payload_cnt3/1 -> Relational3/2
  Constant2/1 -> Relational3/1
  [loop_in_valid] -> Logical10/1
  Delay20/1 -> Logical10/2
  [gbe_in_valid] -> Logical7/1
  [gbe_out_sel] -> Delay6/1
  posedge6/1 -> Logical11/2, Logical17/1
  Logical11/1 -> rd_pkt0/1(start)
  rd_pkt0/1(out) -> [loop_out_sel], negedge/1
  [pkt_rdy] -> Inverter3/1
  Inverter3/1 -> Logical17/2
  Logical17/1 -> rd_pkt1/1(start)
  rd_pkt1/1(out) -> negedge1/1, [gbe_out_sel]
  [gbe_in_valid] -> Register2/3, Register2/1, payload_cnt1/1
  [loop_in_valid] -> Register3/3, Register3/1, payload_cnt3/1
  negedge/1 -> [loop_out_done]
  negedge1/1 -> [gbe_out_done]
  [loop_eof] -> Register3/2, Logical20/1
  [gbe_eof] -> Register2/2, Logical8/1
  [gbe_out_done] -> Delay3/1
  Logical8/1 -> payload_cnt1/2
  Logical20/1 -> payload_cnt3/2
  Relational2/1 -> [gbe_stutter_rd]
  Relational3/1 -> [loop_stutter_rd]
  Inverter8/1 -> Logical12/2
  [gbe_eof] -> Inverter8/1
  [loop_out_done] -> Delay4/1
  Inverter9/1 -> Logical21/2
  [loop_eof] -> Inverter9/1
  Logical12/1 -> [gbe_pkt_oversize]
  Logical21/1 -> [loop_pkt_oversize]
  Slice6/1 -> [loop_timeout]
  Slice10/1 -> [gbe_timeout]
  [rst] -> Logical16/2
  [rst] -> Logical4/2
  [gbe_timeout] -> Logical16/1
  [loop_timeout] -> Logical4/1
  [gbe_pkt_oversize] -> Logical16/3
  [loop_pkt_oversize] -> Logical4/3
  [gbe_eof] -> Register1/2, payload_cnt2/1
  payload_cnt2/1 -> Relational4/2
  Constant3/1 -> Relational4/1
  Relational4/1 -> [gbe_stutter_flush]
  Register1/1 -> payload_cnt2/2, [gbe_rst]
  [loop_eof] -> payload_cnt4/1, Register4/2
  payload_cnt4/1 -> Relational5/2
  Constant4/1 -> Relational5/1
  Register4/1 -> payload_cnt4/2, [loopback_rst]
  Relational5/1 -> [loop_stutter_flush]
  [gbe_out_sel] -> Logical13/1
  [gbe_stutter_rd] -> Logical13/2
  [gbe_stutter_flush] -> Logical13/3
  [loop_out_sel] -> Logical3/1
  [loop_stutter_rd] -> Logical3/2
  [loop_stutter_flush] -> Logical3/3
  Inverter2/1 -> Logical22/1
  Convert9/1 -> Inverter2/1
  [gbe_rst] -> Inverter11/1
  Inverter11/1 -> Logical22/2
  Inverter12/1 -> Logical23/2
  Logical23/1 -> Logical20/2, [loop_rd_hdr]
  Inverter4/1 -> Logical23/1
  [loopback_rst] -> Inverter12/1
  Gateway Out19/1 -> mcnt_verify/8
  Gateway Out18/1 -> mcnt_verify/9
  [loop_data_rdy] -> Gateway Out24/1
  [gbe_data_rdy] -> Gateway Out25/1
  [loop_rd_hdr] -> Gateway Out26/1
  [gbe_rd_hdr] -> Gateway Out16/1
  [loop_eof] -> Gateway Out19/1
  [gbe_eof] -> Gateway Out18/1
  Delay3/1 -> Logical12/1
  Delay4/1 -> Logical21/1
  Gateway Out20/1 -> supervisor_debug/8
  Gateway Out23/1 -> supervisor_debug/9
  [loop_err] -> Gateway Out8/1
  [gbe_err] -> Gateway Out20/1
  Gateway Out30/1 -> supervisor_debug/10
  [gbe_out_sel] -> Inverter5/1
  [loop_out_sel] -> Inverter13/1
  Inverter5/1 -> Delay13/1
  Inverter13/1 -> Delay15/1
  [loop_data_rdy] -> Logical26/3
  [gbe_data_rdy] -> Logical26/4
  Logical26/1 -> posedge6/1
  [loop_ack] -> Gateway Out23/1
  [gbe_ack] -> Gateway Out30/1
  [loop_rd_hdr] -> Inverter15/1
  [gbe_rd_hdr] -> Inverter14/1
  Inverter15/1 -> Logical26/5
  Inverter14/1 -> Logical26/6
  Delay8/1 -> Mux2/1
  Delay9/1 -> Mux6/1
  [loop_out_sel] -> Delay9/1
  Delay10/1 -> Mux3/1
  Delay7/1 -> Mux1/1
  [gbe_out_sel] -> Logical25/1
  [loop_out_sel] -> Logical25/2
  Logical25/1 -> [logic_error]
  Gateway Out31/1 -> supervisor_debug/11
  [logic_error] -> Gateway Out31/1
  Gateway Out32/1 -> mux_debug1/3
  Gateway Out41/1 -> mux_debug1/1
  Gateway Out40/1 -> mux_debug1/2
  Gateway Out35/1 -> mux_debug1/4
  Gateway Out36/1 -> mux_debug1/5
  Gateway Out37/1 -> mux_debug1/6
  Gateway Out42/1 -> mux_debug1/7
  Gateway Out33/1 -> mux_debug1/8
  Gateway Out34/1 -> mux_debug1/9
  Gateway Out38/1 -> mux_debug1/10
  Gateway Out39/1 -> mux_debug1/11
  [loop_in_valid] -> Gateway Out41/1
  [gbe_in_valid] -> Gateway Out40/1
  [loop_eof] -> Gateway Out36/1
  [gbe_eof] -> Gateway Out37/1
  [gbe_out_sel] -> Delay12/1
  [loop_out_sel] -> Delay11/1
  [loop_stutter_rd] -> Delay17/1
  [gbe_stutter_rd] -> Delay18/1
  Delay11/1 -> Gateway Out32/1
  Delay12/1 -> Gateway Out35/1
  Delay17/1 -> Gateway Out42/1
  Delay18/1 -> Gateway Out33/1
  [loop_data_rdy] -> Gateway Out34/1
  [gbe_data_rdy] -> Gateway Out38/1
  Gateway Out43/1 -> mux_debug1/12
  [loop_rd_hdr] -> Gateway Out39/1
  [gbe_rd_hdr] -> Gateway Out43/1
  Delay13/1 -> Logical26/1
  Delay15/1 -> Logical26/2
  Inverter10/1 -> Logical26/7
  Inverter1/1 -> Logical26/8
  [loopback_rst] -> Inverter10/1
  [gbe_rst] -> Inverter1/1
  [loop_eof] -> rd_pkt0/2(eof_rx)
  [gbe_eof] -> rd_pkt1/2(eof_rx)
  [gbe_din] -> Mux/2
  [loop_din] -> Mux/3
  Logical10/1 -> Mux1/3
  Logical7/1 -> Mux1/2
  [gbe_eof] -> Mux2/2
  [loop_eof] -> Mux2/3
  [gbe_hdr] -> Mux6/2
  [loop_hdr] -> Mux6/3
  [gbe_ip] -> Mux3/2
  [loop_ip] -> Mux3/3
  Delay6/1 -> Logical7/2
  rd_pkt1/2(pkt_size_err) -> [gbe_pkt_undersize_err]
  rd_pkt0/2(pkt_size_err) -> [loop_pkt_undersize_err]
  Logical1/1 -> Counter1/2, [loop_err]
  [loop_pkt_undersize_err] -> Logical1/1
  Logical6/1 -> Counter3/2, [gbe_err]
  [gbe_pkt_undersize_err] -> Logical6/1
  [loop_err] -> Logical18/1
  [gbe_err] -> Logical18/2
